simulink model "flc_pid"  (R2014a)
settings: Solver=ode45  StartTime=0.0  StopTime=10  RelTol=1e-3
libraries: fuzblock x1, simulink x1
settings Model: Creator=krish  LastModifiedBy=krish
settings DebuggingCC: SolverPrmCheckMsg=none

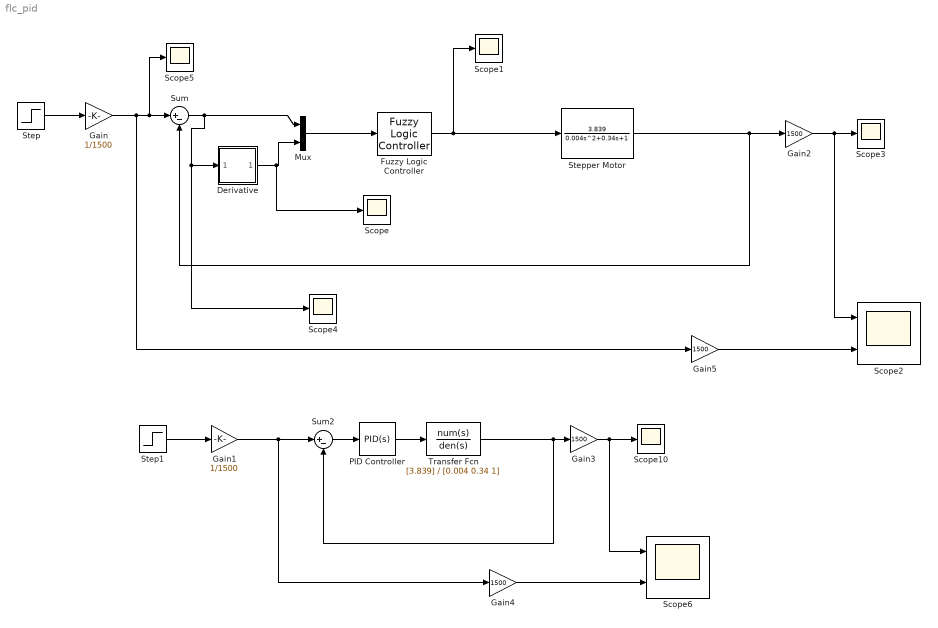
== system flc_pid ==
  Derivative : Subsystem
  Fuzzy Logic Controller : fuzblock/Fuzzy Logic  Controller  fis='flc_pid2.fis'
  Gain : Gain  Gain=1/1500
  Gain1 : Gain  Gain=1/1500
  Gain{2..5} (4 alike) : Gain  Gain=1500
  Mux : Mux  Inputs=2
  PID Controller : simulink/Continuous/PID Controller  Controller=PID  TimeDomain=Continuous-time  SampleTime=1  IntegratorMethod=Forward Euler  FilterMethod=Forward Euler  Form=Parallel  P=0.200774918416971  I=1.23789446397102  D=-0.0190825718357155  N=10.5213762665468  InitialConditionSource=internal  InitialConditionForIntegrator=0  InitialConditionForFilter=0  ExternalReset=none  LimitOutput=off  UpperSaturationLimit=inf  LowerSaturationLimit=-inf  LinearizeAsGain=on  AntiWindupMode=none  Kb=1  TrackingMode=off  Kt=1  PParamMin=[]  PParamMax=[]  IParamMin=[]  IParamMax=[]  DParamMin=[]  DParamMax=[]  NParamMin=[]  NParamMax=[]  KbParamMin=[]  KbParamMax=[]  KtParamMin=[]  KtParamMax=[]  POutMin=[]  POutMax=[]  IOutMin=[]  IOutMax=[]  DOutMin=[]  DOutMax=[]  NOutMin=[]  NOutMax=[]  KbOutMin=[]  KbOutMax=[]  KtOutMin=[]  KtOutMax=[]  IntegratorOutMin=[]  IntegratorOutMax=[]  FilterOutMin=[]  FilterOutMax=[]  SumOutMin=[]  SumOutMax=[]  SumI1OutMin=[]  SumI1OutMax=[]  SumI2OutMin=[]  SumI2OutMax=[]  SumI3OutMin=[]  SumI3OutMax=[]  SumDOutMin=[]  SumDOutMax=[]  SaturationOutMin=[]  SaturationOutMax=[]  IntegratorContinuousStateAttributes=''  IntegratorStateMustResolveToSignalObject=off  IntegratorRTWStateStorageClass=Auto  FilterContinuousStateAttributes=''  FilterStateMustResolveToSignalObject=off  FilterRTWStateStorageClass=Auto
  Scope{,1,3..5,10} (6 alike) : Scope
      Scope1 settings: TimeRange=0.4499999999999993  YMin=0  YMax=0.8
      Scope10 settings: SaveName=ScopeData10
      Scope3 settings: SaveName=ScopeData3
      Scope4 settings: SaveName=ScopeData4
      Scope5 settings: YMin=0.855  YMax=0.945  SaveName=ScopeData5
  Scope2 : Scope  NumInputPorts=2
      settings: TimeRange=10  YMin=0~800  YMax=60000~1500  SaveName=ScopeData2
  Scope6 : Scope  NumInputPorts=2
      settings: TimeRange=10  YMin=1449.978~1449.999999825  YMax=1449.998~1450.000000175  SaveName=ScopeData6
  Step : Step  Time=5  Before=800  After=1450  SampleTime=0.001  VectorParams1D=off
  Step1 : Step  Time=5  Before=800  After=1450  SampleTime=0  VectorParams1D=off  ZeroCross=off
  "Stepper Motor " : TransferFcn  Numerator=[3.839]  Denominator=[0.004 0.34 1]
  Sum : Sum  Inputs=|+-
  Sum2 : Sum  Inputs=|+-
  Transfer Fcn : TransferFcn  Numerator=[3.839]  Denominator=[0.004 0.34 1]
  wires:
  Sum/1 -> Derivative/1(in_1), Scope4/1, Mux/1
  "Stepper Motor "/1 -> Gain2/1, Sum/2
  Mux/1 -> Fuzzy Logic Controller/1
  Fuzzy Logic Controller/1 -> "Stepper Motor "/1, Scope1/1
  Step/1 -> Gain/1
  Sum2/1 -> PID Controller/1
  PID Controller/1 -> Transfer Fcn/1
  Transfer Fcn/1 -> Sum2/2, Gain3/1
  Step1/1 -> Gain1/1
  Gain/1 -> Gain5/1, Sum/1, Scope5/1
  Gain1/1 -> Gain4/1, Sum2/1
  Gain2/1 -> Scope2/1, Scope3/1
  Gain3/1 -> Scope6/1, Scope10/1
  Gain4/1 -> Scope6/2
  Gain5/1 -> Scope2/2
  Derivative/1(out_1) -> Scope/1, Mux/2

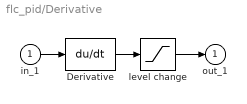
== system flc_pid/Derivative ==
  in_1 : Inport
  Derivative : Derivative
  level change : Saturate  UpperLimit=1  LowerLimit=-1
  out_1 : Outport
  wires:
  in_1/1 -> Derivative/1
  level change/1 -> out_1/1
  Derivative/1 -> level change/1
